simulink model "StateDiagram2"  (R2025b)
settings: Solver=FixedStepAuto  StartTime=0.0  StopTime=Inf  RelTol=1e-3
settings Model: Creator=Soochan Kim  LastModifiedBy=Soochan Kim
settings OptimizationCC: BlockReduction=off  ConditionallyExecuteInputs=off  DefaultParameterBehavior=Inlined  OptimizeBlockIOStorage=off  OptimizeDataStoreBuffers=off  BusAssignmentInplaceUpdate=off
settings DebuggingCC: AlgebraicLoopMsg=error  SFUnexpectedBacktrackingDiag=warning  SFNoUnconditionalDefaultTransitionDiag=warning
settings HardwareCC: ProdBitPerPointer=32.0  ProdBitPerSizeT=32.0  ProdBitPerPtrDiffT=32.0  ProdLargestAtomicFloat=None  ProdIntDivRoundTo=Undefined  ProdEndianess=Unspecified  ProdWordSize=32.0  ProdHWDeviceType=ASIC/FPGA->ASIC/FPGA  TargetBitPerPointer=64.0  TargetBitPerSizeT=64.0  TargetBitPerPtrDiffT=64.0  TargetLongLongMode=on  TargetIntDivRoundTo=Zero  TargetEndianess=LittleEndian  TargetWordSize=64.0  TargetHWDeviceType=Custom Processor->MATLAB Host Computer  ProdEqTarget=off
settings RTWCC: GenCodeOnly=on  GenerateReport=on  BuildConfiguration=Debug  LaunchReport=on
settings CodeAppCC: ForceParamTrailComments=on  MATLABSourceComments=on  EnableCustomComments=on
settings GRTTargetCC: MultiInstanceErrorCode=Warning  CombineSignalStateStructs=on  SupportVariableSizeSignals=on

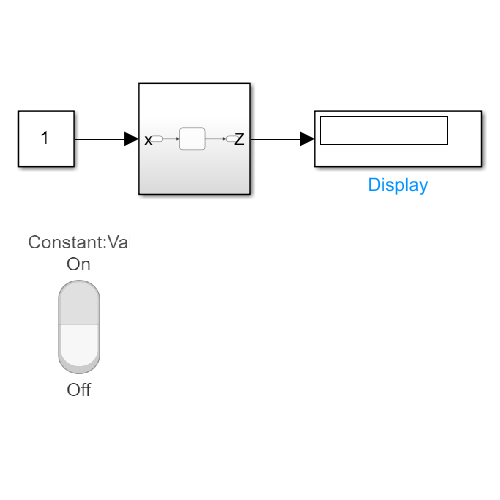
[thumbnail: Simulink's stored preview of the top-level diagram]
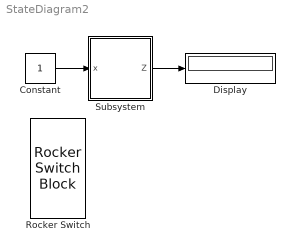
== system StateDiagram2 ==
  Constant : Constant  OutDataTypeStr=boolean
  Display : Display
  Rocker Switch : RockerSwitchBlock
  Subsystem : Subsystem
  wires:
  Constant/1 -> Subsystem/1(x)
  Subsystem/1(Z) -> Display/1

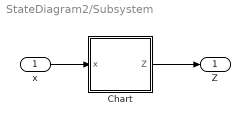
== system StateDiagram2/Subsystem ==
  x : Inport
  Chart : Stateflow chart  TreatAsAtomicUnit=on
  Z : Outport  OutDataTypeStr=boolean
  wires:
  x/1 -> Chart/1(x)
  Chart/1(Z) -> Z/1

== stateflow chart StateDiagram2/Subsystem/Chart ==
  settings: stateMachineType=MOORE_MACHINE  executeAtInitialization=1  initializeOutput=1
  state S0
    Z=false;
  state S3
    Z=true;
  state S1
    Z=true;
  state S2
    Z=false;
  (default) -> S0
  S0 -> S1 [order 2] : [x==1]
  S0 -> S3 [order 1] : [x==0]
  S1 -> S0 [order 1] : [x==0]
  S3 -> S1 [order 2] : [x==1]
  S3 -> S2 [order 1] : [x==0]
  S1 -> S2 [order 2] : [x==1]
  S2 -> S1 [order 1] : [x==0]
  S2 -> S2 [order 2] : [x==1]
  data: x input; Z output boolean
